simulink model "EMPlanner_cs"  (R2023a)
settings: Solver=ode5  StartTime=0.0  StopTime=60  FixedStep=1/1000  RelTol=1e-3
PreLoadFcn:
  | mbxruntime.callbacks.PreLoadFcn(bdroot);
PostLoadFcn:
  | mbxruntime.callbacks.PostLoadFcn(bdroot);
InitFcn:
  | mbxruntime.callbacks.InitFcn(bdroot);
StartFcn:
  | mbxruntime.callbacks.StartFcn(bdroot);
StopFcn:
  | mbxruntime.callbacks.StopFcn(bdroot);
model workspace: external: MAT-File .\EMPlanner_cs_hws.mat (data not in the file)
values from neighbouring files (symbols this model uses):
  c_factor = 43.75    [emplanner_init.m]
  cf = -64276.3    [emplanner_init.m]
  cr = -64276.3    [emplanner_init.m]
  KD_PID_distance = 0.0    (= 0)    [emplanner_init.m]
  KD_PID_speed = 0    [emplanner_init.m]
  KI_PID_distance = 0.0    (= 0)    [emplanner_init.m]
  KI_PID_speed = 0    [emplanner_init.m]
  KP_PID_distance = 0.5    [emplanner_init.m]
  KP_PID_speed = 1.8    [emplanner_init.m]
  la = 0.5989    [emplanner_init.m]
  lb = 1.1979-0.5989    (= 0.599)    [emplanner_init.m]
  LQR_K1 = k(:,1)'    [emplanner_init.m]
  LQR_K2 = k(:,2)'    [emplanner_init.m]
  LQR_K3 = k(:,3)'    [emplanner_init.m]
  LQR_K4 = k(:,4)'    [emplanner_init.m]
  m = 375.8    [emplanner_init.m]
  vx_break_point = zeros(1,5000)    [emplanner_init.m]
undefined symbols (not defined in the file or in its folder): aubr, DiscIntNeverNeededParam, EMPlanner_cs_27357ced727cddc2, EMPlanner_cs_3a309230b46bf2dd, EMPlanner_cs_4725e6271df7126f, EMPlanner_cs_7cd0898d5750b5ce, EMPlanner_cs_9531ed1ae61b92f2, EMPlanner_cs_Box_10_Dynamics_Empty_STATE_Box_10_Pitch0, EMPlanner_cs_Box_10_Dynamics_Empty_STATE_Box_10_Roll0, EMPlanner_cs_Box_10_Dynamics_Empty_STATE_Box_10_x0, EMPlanner_cs_Box_10_Dynamics_Empty_STATE_Box_10_y0, EMPlanner_cs_Box_10_Dynamics_Empty_STATE_Box_10_Yaw0, EMPlanner_cs_Box_10_Dynamics_Empty_STATE_Box_10_z0, EMPlanner_cs_Box_11_Dynamics_Empty_STATE_Box_11_Pitch0, EMPlanner_cs_Box_11_Dynamics_Empty_STATE_Box_11_Roll0, EMPlanner_cs_Box_11_Dynamics_Empty_STATE_Box_11_x0, EMPlanner_cs_Box_11_Dynamics_Empty_STATE_Box_11_y0, EMPlanner_cs_Box_11_Dynamics_Empty_STATE_Box_11_Yaw0, EMPlanner_cs_Box_11_Dynamics_Empty_STATE_Box_11_z0, EMPlanner_cs_Box_12_Dynamics_Empty_STATE_Box_12_Pitch0, EMPlanner_cs_Box_12_Dynamics_Empty_STATE_Box_12_Roll0, EMPlanner_cs_Box_12_Dynamics_Empty_STATE_Box_12_x0, EMPlanner_cs_Box_12_Dynamics_Empty_STATE_Box_12_y0, EMPlanner_cs_Box_12_Dynamics_Empty_STATE_Box_12_Yaw0, EMPlanner_cs_Box_12_Dynamics_Empty_STATE_Box_12_z0, EMPlanner_cs_Box_1_Path_pathUniqueID, EMPlanner_cs_Box_1_SpeedProfile_speedProfileUniqueID, EMPlanner_cs_Box_2_Path_pathUniqueID, EMPlanner_cs_Box_2_SpeedProfile_speedProfileUniqueID, EMPlanner_cs_Box_3_Path_pathUniqueID, EMPlanner_cs_Box_3_SpeedProfile_speedProfileUniqueID, EMPlanner_cs_Box_4_Path_pathUniqueID, EMPlanner_cs_Box_4_SpeedProfile_speedProfileUniqueID, EMPlanner_cs_Box_5_Dynamics_Empty_STATE_Box_5_Pitch0, EMPlanner_cs_Box_5_Dynamics_Empty_STATE_Box_5_Roll0, EMPlanner_cs_Box_5_Dynamics_Empty_STATE_Box_5_x0, EMPlanner_cs_Box_5_Dynamics_Empty_STATE_Box_5_y0, EMPlanner_cs_Box_5_Dynamics_Empty_STATE_Box_5_Yaw0, EMPlanner_cs_Box_5_Dynamics_Empty_STATE_Box_5_z0, EMPlanner_cs_Box_6_Path_pathUniqueID, EMPlanner_cs_Box_6_SpeedProfile_speedProfileUniqueID, EMPlanner_cs_Box_7_Dynamics_Empty_STATE_Box_7_Pitch0, EMPlanner_cs_Box_7_Dynamics_Empty_STATE_Box_7_Roll0, EMPlanner_cs_Box_7_Dynamics_Empty_STATE_Box_7_x0, EMPlanner_cs_Box_7_Dynamics_Empty_STATE_Box_7_y0, EMPlanner_cs_Box_7_Dynamics_Empty_STATE_Box_7_Yaw0, EMPlanner_cs_Box_7_Dynamics_Empty_STATE_Box_7_z0, EMPlanner_cs_Box_8_Dynamics_Empty_STATE_Box_8_Pitch0, EMPlanner_cs_Box_8_Dynamics_Empty_STATE_Box_8_Roll0, EMPlanner_cs_Box_8_Dynamics_Empty_STATE_Box_8_x0, EMPlanner_cs_Box_8_Dynamics_Empty_STATE_Box_8_y0, EMPlanner_cs_Box_8_Dynamics_Empty_STATE_Box_8_Yaw0, EMPlanner_cs_Box_8_Dynamics_Empty_STATE_Box_8_z0, EMPlanner_cs_Box_9_Dynamics_Empty_STATE_Box_9_Pitch0, EMPlanner_cs_Box_9_Dynamics_Empty_STATE_Box_9_Roll0, EMPlanner_cs_Box_9_Dynamics_Empty_STATE_Box_9_x0, EMPlanner_cs_Box_9_Dynamics_Empty_STATE_Box_9_y0, EMPlanner_cs_Box_9_Dynamics_Empty_STATE_Box_9_Yaw0, EMPlanner_cs_Box_9_Dynamics_Empty_STATE_Box_9_z0, EMPlanner_cs_dca7ae789a013f83 ... (+7)
libraries: PreScanSimulinkLibrary x16, Solver_SF x1
(part 7 of 10)

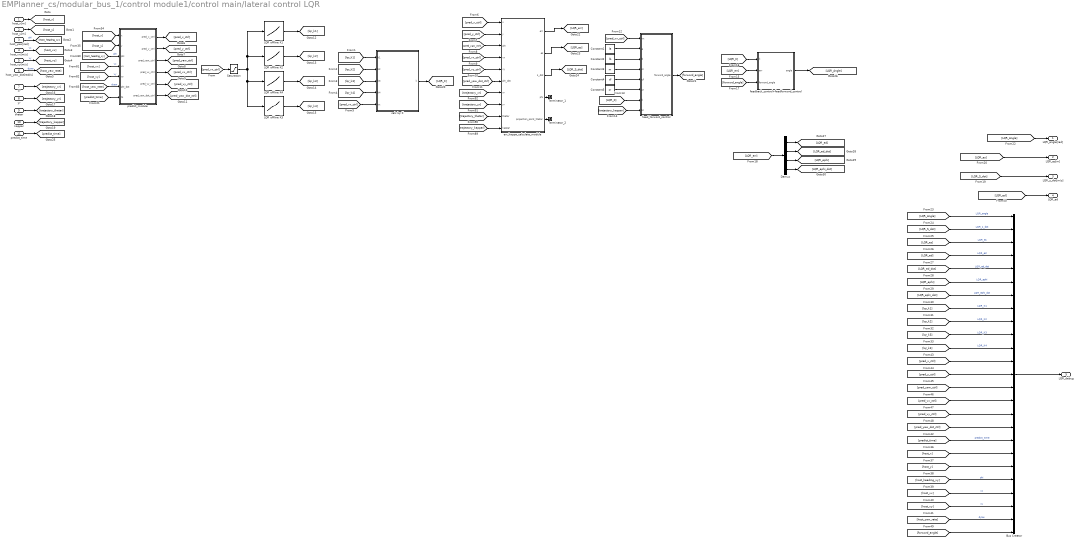
== system EMPlanner_cs/modular_bus_1/control module1/control main/lateral control LQR ==
  host_x[m] : Inport
  host_y[m] : Inport  Port=2
  host_yaw[rad] : Inport  Port=3
  host_vx[m/s] : Inport  Port=4
  host_vy[m/s] : Inport  Port=5
  host_yaw_dot[rad/s] : Inport  Port=6
  xr : Inport  Port=7
  yr : Inport  Port=8
  thetar : Inport  Port=9
  kappar : Inport  Port=10
  predict_time : Inport  Port=11
  Bus Creator : BusCreator  Inputs=25
  Constant1 : Constant  Value=la
  Constant2 : Constant  Value=lb
  Constant3 : Constant  Value=m
  Constant4 : Constant  Value=cf
  Constant5 : Constant  Value=cr
  Demux : Demux
  LQR offline K1 : Lookup_n-D  NumberOfTableDimensions=1  BreakpointsForDimension1=vx_break_point  Table=LQR_K1  InternalRulePriority=Speed  RndMeth=Simplest
  LQR offline K2 : Lookup_n-D  NumberOfTableDimensions=1  BreakpointsForDimension1=vx_break_point  Table=LQR_K2  InternalRulePriority=Speed  RndMeth=Simplest
  LQR offline K3 : Lookup_n-D  NumberOfTableDimensions=1  BreakpointsForDimension1=vx_break_point  Table=LQR_K3  InternalRulePriority=Speed  RndMeth=Simplest
  LQR offline K4 : Lookup_n-D  NumberOfTableDimensions=1  BreakpointsForDimension1=vx_break_point  Table=LQR_K4  InternalRulePriority=Speed  RndMeth=Simplest
  Saturation : Saturate  UpperLimit=50  LowerLimit=0
  Terminator_1 : Terminator
  Terminator_2 : Terminator
  calc lqr K : MATLAB Function  TreatAsAtomicUnit=on
  err_kappa_calculate_module : MATLAB Function  TreatAsAtomicUnit=on
  feed_forword_control : MATLAB Function  TreatAsAtomicUnit=on
  feedback_control+feedforword_control : MATLAB Function  TreatAsAtomicUnit=on
  predict_module : MATLAB Function  TreatAsAtomicUnit=on
  LQR_angle[rad] : Outport  VectorParamsAs1DForOutWhenUnconnected=off
  LQR_es[m] : Outport  Port=2  VectorParamsAs1DForOutWhenUnconnected=off
  LQR_s_dot[m/s] : Outport  Port=3  VectorParamsAs1DForOutWhenUnconnected=off
  LQR_ed : Outport  Port=4  VectorParamsAs1DForOutWhenUnconnected=off
  LQR_debug : Outport  Port=5  VectorParamsAs1DForOutWhenUnconnected=off
  wires:
  err_kappa_calculate_module/5(projection_point_thetar) -> Terminator_2/1
  err_kappa_calculate_module/4(phi) -> Terminator_1/1
  [LQR_ed] -> LQR_ed/1
  [forword_angle] -> Bus Creator/25
  [host_yaw_rate] -> Bus Creator/24  "dyaw"
  [host_vy] -> Bus Creator/23  "vy"
  [host_vx] -> Bus Creator/22  "vx"
  [host_heading_xy] -> Bus Creator/21  "phi"
  [host_y] -> Bus Creator/20
  [host_x] -> Bus Creator/19
  [predict_time] -> Bus Creator/18  "predict_time"
  [pred_yaw_dot_ctrl] -> Bus Creator/17
  [pred_vy_ctrl] -> Bus Creator/16
  [pred_vx_ctrl] -> Bus Creator/15
  [pred_yaw_ctrl] -> Bus Creator/14
  [pred_y_ctrl] -> Bus Creator/13
  [pred_x_ctrl] -> Bus Creator/12
  [lqr_k4] -> Bus Creator/11  "LQR_K4"
  [lqr_k3] -> Bus Creator/10  "LQR_K3"
  [lqr_k2] -> Bus Creator/9  "LQR_K2"
  [lqr_k1] -> Bus Creator/8  "LQR_K1"
  [LQR_ephi_dot] -> Bus Creator/7  "LQR_ephi_dot"
  [LQR_ephi] -> Bus Creator/6  "LQR_ephi"
  [LQR_ed_dot] -> Bus Creator/5  "LQR_ed_dot"
  [LQR_ed] -> Bus Creator/4  "LQR_ed"
  Demux/4 -> [LQR_ephi_dot]
  Demux/3 -> [LQR_ephi]
  Demux/2 -> [LQR_ed_dot]
  Demux/1 -> [LQR_ed]
  [LQR_es] -> Bus Creator/3  "LQR_es"
  [LQR_S_dot] -> Bus Creator/2  "LQR_s_dot"
  [LQR_Angle] -> Bus Creator/1  "LQR_angle"
  [LQR_Angle] -> LQR_angle[rad]/1
  feedback_control+feedforword_control/1(angle) -> [LQR_Angle]
  Bus Creator/1 -> LQR_debug/1
  predict_time/1 -> [predict_time]
  Saturation/1 -> LQR offline K1/1, LQR offline K2/1, LQR offline K4/1, LQR offline K3/1
  [LQR_es] -> LQR_es[m]/1
  [LQR_S_dot] -> LQR_s_dot[m/s]/1
  err_kappa_calculate_module/3(s_dot) -> [LQR_S_dot]
  err_kappa_calculate_module/2(es) -> [LQR_es]
  [LQR_err] -> Demux/1
  [forword_angle] -> feedback_control+feedforword_control/3(forword_angle)
  [LQR_K] -> feedback_control+feedforword_control/1(k)
  [LQR_err] -> feedback_control+feedforword_control/2(err)
  err_kappa_calculate_module/1(err) -> [LQR_err]
  feed_forword_control/1(forword_angle) -> [forword_angle]
  [trajectory_kappar] -> feed_forword_control/8(kr)
  [LQR_K] -> feed_forword_control/7(k)
  calc lqr K/1(k) -> [LQR_K]
  Constant5/1 -> feed_forword_control/6(cr)
  Constant4/1 -> feed_forword_control/5(cf)
  Constant3/1 -> feed_forword_control/4(m)
  Constant2/1 -> feed_forword_control/3(b)
  Constant1/1 -> feed_forword_control/2(a)
  [pred_vx_ctrl] -> feed_forword_control/1(vx)
  [trajectory_thetar] -> err_kappa_calculate_module/9(thetar)
  [trajectory_kappar] -> err_kappa_calculate_module/10(kappar)
  [trajectory_yr] -> err_kappa_calculate_module/8(yr)
  [trajectory_xr] -> err_kappa_calculate_module/7(xr)
  kappar/1 -> [trajectory_kappar]
  thetar/1 -> [trajectory_thetar]
  yr/1 -> [trajectory_yr]
  xr/1 -> [trajectory_xr]
  [pred_yaw_dot_ctrl] -> err_kappa_calculate_module/6(phi_dot)
  [pred_vy_ctrl] -> err_kappa_calculate_module/5(vy)
  [pred_vx_ctrl] -> err_kappa_calculate_module/4(vx)
  [pred_yaw_ctrl] -> err_kappa_calculate_module/3("phi ")
  [pred_y_ctrl] -> err_kappa_calculate_module/2(y)
  [pred_x_ctrl] -> err_kappa_calculate_module/1(x)
  [lqr_k1] -> calc lqr K/1(k1)
  [lqr_k2] -> calc lqr K/2(k2)
  [lqr_k3] -> calc lqr K/3(k3)
  [lqr_k4] -> calc lqr K/4(k4)
  [pred_vx_ctrl] -> calc lqr K/5(vx)
  LQR offline K3/1 -> [lqr_k4]
  LQR offline K4/1 -> [lqr_k3]
  LQR offline K2/1 -> [lqr_k2]
  LQR offline K1/1 -> [lqr_k1]
  [pred_vx_ctrl] -> Saturation/1
  predict_module/6(pred_yaw_dot_ctrl) -> [pred_yaw_dot_ctrl]
  predict_module/5(pred_vy_ctrl) -> [pred_vy_ctrl]
  predict_module/4(pred_vx_ctrl) -> [pred_vx_ctrl]
  predict_module/3(pred_yaw_ctrl) -> [pred_yaw_ctrl]
  predict_module/2(pred_y_ctrl) -> [pred_y_ctrl]
  predict_module/1(pred_x_ctrl) -> [pred_x_ctrl]
  host_yaw_dot[rad/s]/1 -> [host_yaw_rate]  "dyaw"
  host_vy[m/s]/1 -> [host_vy]  "vy"
  host_vx[m/s]/1 -> [host_vx]  "vx"
  host_yaw[rad]/1 -> [host_heading_xy]  "phi"
  host_y[m]/1 -> [host_y]
  host_x[m]/1 -> [host_x]
  [predict_time] -> predict_module/7(ts)
  [host_heading_xy] -> predict_module/3(phi)  "phi"
  [host_y] -> predict_module/2(y)
  [host_vx] -> predict_module/4(vx)  "vx"
  [host_yaw_rate] -> predict_module/6(phi_dot)  "dyaw"
  [host_x] -> predict_module/1(x)
  [host_vy] -> predict_module/5(vy)  "vy"

== system EMPlanner_cs/modular_bus_1/control module1/control main/longitudinal control double PID ==
  s_err[m] : Inport
  speed_desire[m/s] : Inport  Port=2
  accelerate desire[m/s^2] : Inport  Port=3
  host_speed[m/s] : Inport  Port=4
  host_s_dot[m/s] : Inport  Port=5
  KP_PID_distance : Inport  Port=6
  KI_PID_distance : Inport  Port=7
  KD_PID_distance : Inport  Port=8
  KP_PID_speed : Inport  Port=9
  KI_PID_speed : Inport  Port=10
  KD_PID_speed : Inport  Port=11
  2-D Lookup Table : Lookup_n-D  BreakpointsForDimension1=vubr  BreakpointsForDimension2=aubr  Table=tablebr  InternalRulePriority=Speed  RndMeth=Simplest
      settings: InputPortMap=u0,u1
  Add : Sum  Inputs=++-
  Add1 : Sum
  Bus Creator : BusCreator  Inputs=9
  Discrete Filter : DiscreteFilter
  MATLAB Function1 : MATLAB Function  TreatAsAtomicUnit=on
  Saturation : Saturate  UpperLimit=45  LowerLimit=-45
  Saturation1 : Saturate  UpperLimit=5  LowerLimit=-8
  discrete pid distance : Subsystem
  discrete pid speed : Subsystem
  throttle : Outport
  brake : Outport  Port=2
  longitudinal_debug : Outport  Port=3
  wires:
  discrete pid distance/1(pid_out) -> Add/1
  [KD_PID_speed] -> discrete pid speed/4(kd)
  [KI_PID_speed] -> discrete pid speed/3(ki)
  [KP_PID_speed] -> discrete pid speed/2(kp)
  [KD_PID_distance] -> discrete pid distance/4(kd)
  [KI_PID_distance] -> discrete pid distance/3(ki)
  [KP_PID_distance] -> discrete pid distance/2(kp)
  Discrete Filter/1 -> discrete pid distance/1(err)
  Bus Creator/1 -> longitudinal_debug/1
  [host_s_dot] -> Bus Creator/9  "host_s_dot"
  [s_err] -> Bus Creator/8  "s_err"
  [host_speed] -> Bus Creator/7  "host_speed"
  [KD_PID_speed] -> Bus Creator/6  "KD_PID_speed"
  [KI_PID_speed] -> Bus Creator/5  "KI_PID_speed"
  [KP_PID_speed] -> Bus Creator/4  "KP_PID_speed"
  [KD_PID_distance] -> Bus Creator/3  "KD_PID_distance"
  [KI_PID_distance] -> Bus Creator/2  "KI_PID_distance"
  [KP_PID_distance] -> Bus Creator/1  "KP_PID_distance"
  MATLAB Function1/2(brake) -> brake/1
  MATLAB Function1/1(throttle) -> throttle/1
  [host_speed] -> 2-D Lookup Table/1
  [host_s_dot] -> Add/3
  host_s_dot[m/s]/1 -> [host_s_dot]
  Saturation1/1 -> 2-D Lookup Table/2
  Add1/1 -> Saturation1/1
  [accelerate_desire] -> Add1/2
  discrete pid speed/1(pid_out) -> Add1/1
  Saturation/1 -> discrete pid speed/1(err)
  Add/1 -> Saturation/1
  [speed_desire] -> Add/2
  host_speed[m/s]/1 -> [host_speed]
  [s_err] -> Discrete Filter/1
  KD_PID_speed/1 -> [KD_PID_speed]
  KI_PID_speed/1 -> [KI_PID_speed]
  KP_PID_speed/1 -> [KP_PID_speed]
  KD_PID_distance/1 -> [KD_PID_distance]
  KI_PID_distance/1 -> [KI_PID_distance]
  KP_PID_distance/1 -> [KP_PID_distance]
  accelerate desire[m/s^2]/1 -> [accelerate_desire]
  speed_desire[m/s]/1 -> [speed_desire]
  s_err[m]/1 -> [s_err]
  2-D Lookup Table/1 -> MATLAB Function1/1(u)

== system EMPlanner_cs/modular_bus_1/control module1/control main/understeer compensate ==
  LQR_angle : Inport
  lateral err : Inport  Port=2
  Add : Sum  Inputs=+-
  Gain : Gain  Gain=0.01
  Manual Switch : ManualSwitch
  LQR_final_angle : Outport
  wires:
  Gain/1 -> Add/2
  LQR_angle/1 -> Manual Switch/1, Add/1
  Manual Switch/1 -> LQR_final_angle/1
  Add/1 -> Manual Switch/2
  lateral err/1 -> Gain/1

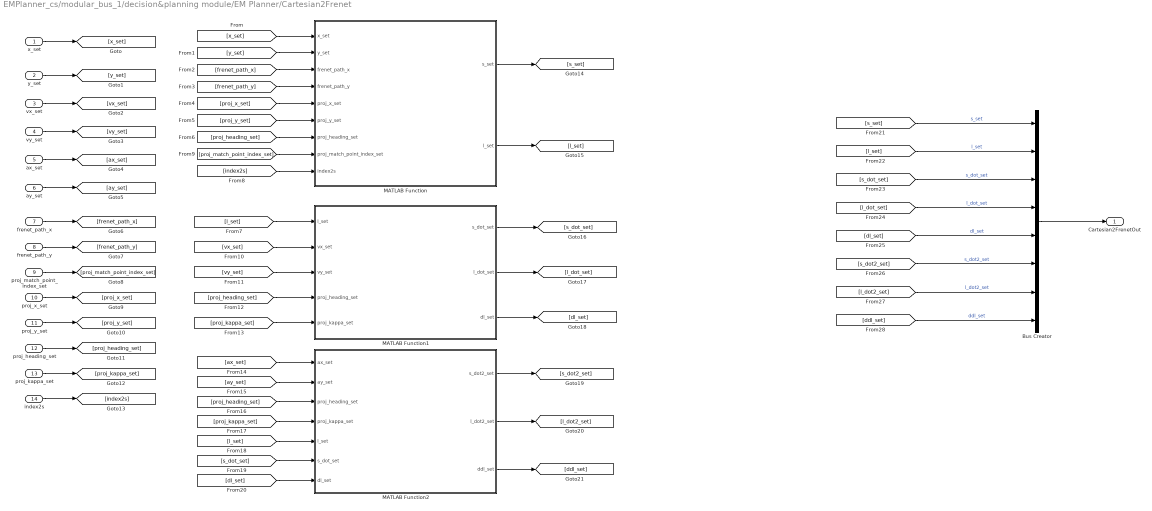
== system EMPlanner_cs/modular_bus_1/decision&planning module/EM Planner/Cartesian2Frenet ==
  x_set : Inport
  y_set : Inport  Port=2
  vx_set : Inport  Port=3
  vy_set : Inport  Port=4
  ax_set : Inport  Port=5
  ay_set : Inport  Port=6
  frenet_path_x : Inport  Port=7
  frenet_path_y : Inport  Port=8
  proj_match_point_index_set : Inport  Port=9
  proj_x_set : Inport  Port=10
  proj_y_set : Inport  Port=11
  proj_heading_set : Inport  Port=12
  proj_kappa_set : Inport  Port=13
  index2s : Inport  Port=14
  Bus Creator : BusCreator  Inputs=8
  MATLAB Function : MATLAB Function  TreatAsAtomicUnit=on
  MATLAB Function1 : MATLAB Function  TreatAsAtomicUnit=on
  MATLAB Function2 : MATLAB Function  TreatAsAtomicUnit=on
  Cartesian2FrenetOut : Outport
  wires:
  Bus Creator/1 -> Cartesian2FrenetOut/1
  [ddl_set] -> Bus Creator/8  "ddl_set"
  [l_dot2_set] -> Bus Creator/7  "l_dot2_set"
  [s_dot2_set] -> Bus Creator/6  "s_dot2_set"
  [dl_set] -> Bus Creator/5  "dl_set"
  [l_dot_set] -> Bus Creator/4  "l_dot_set"
  [s_dot_set] -> Bus Creator/3  "s_dot_set"
  [l_set] -> Bus Creator/2  "l_set"
  [s_set] -> Bus Creator/1  "s_set"
  MATLAB Function2/3(ddl_set) -> [ddl_set]
  MATLAB Function2/2(l_dot2_set) -> [l_dot2_set]
  MATLAB Function2/1(s_dot2_set) -> [s_dot2_set]
  [dl_set] -> MATLAB Function2/7(dl_set)
  [s_dot_set] -> MATLAB Function2/6(s_dot_set)
  MATLAB Function1/3(dl_set) -> [dl_set]
  MATLAB Function1/2(l_dot_set) -> [l_dot_set]
  MATLAB Function1/1(s_dot_set) -> [s_dot_set]
  [l_set] -> MATLAB Function2/5(l_set)
  [proj_kappa_set] -> MATLAB Function2/4(proj_kappa_set)
  [proj_heading_set] -> MATLAB Function2/3(proj_heading_set)
  [ay_set] -> MATLAB Function2/2(ay_set)
  [ax_set] -> MATLAB Function2/1(ax_set)
  [proj_kappa_set] -> MATLAB Function1/5(proj_kappa_set)
  [proj_heading_set] -> MATLAB Function1/4(proj_heading_set)
  [vy_set] -> MATLAB Function1/3(vy_set)
  [vx_set] -> MATLAB Function1/2(vx_set)
  [l_set] -> MATLAB Function1/1(l_set)
  MATLAB Function/2(l_set) -> [l_set]
  MATLAB Function/1(s_set) -> [s_set]
  [index2s] -> MATLAB Function/9(index2s)
  [proj_heading_set] -> MATLAB Function/7(proj_heading_set)
  [proj_y_set] -> MATLAB Function/6(proj_y_set)
  [proj_match_point_index_set] -> MATLAB Function/8(proj_match_point_index_set)
  [proj_x_set] -> MATLAB Function/5(proj_x_set)
  [frenet_path_y] -> MATLAB Function/4(frenet_path_y)
  [frenet_path_x] -> MATLAB Function/3(frenet_path_x)
  [y_set] -> MATLAB Function/2(y_set)
  [x_set] -> MATLAB Function/1(x_set)
  index2s/1 -> [index2s]
  proj_kappa_set/1 -> [proj_kappa_set]
  proj_heading_set/1 -> [proj_heading_set]
  proj_y_set/1 -> [proj_y_set]
  proj_x_set/1 -> [proj_x_set]
  proj_match_point_index_set/1 -> [proj_match_point_index_set]
  frenet_path_y/1 -> [frenet_path_y]
  frenet_path_x/1 -> [frenet_path_x]
  ay_set/1 -> [ay_set]
  ax_set/1 -> [ax_set]
  vy_set/1 -> [vy_set]
  vx_set/1 -> [vx_set]
  y_set/1 -> [y_set]
  x_set/1 -> [x_set]

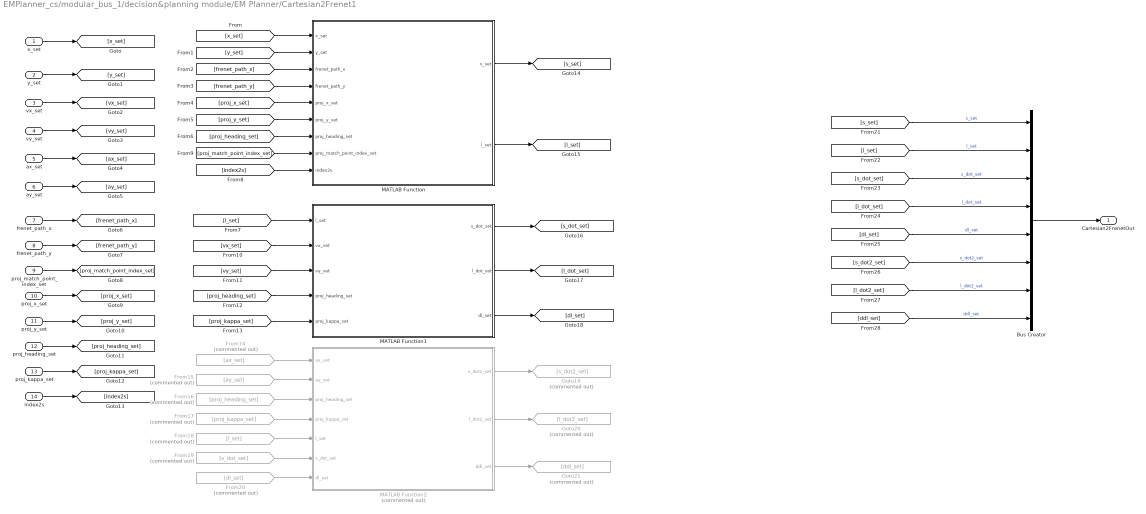
== system EMPlanner_cs/modular_bus_1/decision&planning module/EM Planner/Cartesian2Frenet1 ==
  x_set : Inport
  y_set : Inport  Port=2
  vx_set : Inport  Port=3
  vy_set : Inport  Port=4
  ax_set : Inport  Port=5
  ay_set : Inport  Port=6
  frenet_path_x : Inport  Port=7
  frenet_path_y : Inport  Port=8
  proj_match_point_index_set : Inport  Port=9
  proj_x_set : Inport  Port=10
  proj_y_set : Inport  Port=11
  proj_heading_set : Inport  Port=12
  proj_kappa_set : Inport  Port=13
  index2s : Inport  Port=14
  Bus Creator : BusCreator  Inputs=8
  From14 : From  Commented=on  GotoTag=ax_set
  From15 : From  Commented=on  GotoTag=ay_set
  From16 : From  Commented=on  GotoTag=proj_heading_set
  From17 : From  Commented=on  GotoTag=proj_kappa_set
  From18 : From  Commented=on  GotoTag=l_set
  From19 : From  Commented=on  GotoTag=s_dot_set
  From20 : From  Commented=on  GotoTag=dl_set
  Goto19 : Goto  Commented=on  GotoTag=s_dot2_set
  Goto20 : Goto  Commented=on  GotoTag=l_dot2_set
  Goto21 : Goto  Commented=on  GotoTag=ddl_set
  MATLAB Function : MATLAB Function  TreatAsAtomicUnit=on
  MATLAB Function1 : MATLAB Function  TreatAsAtomicUnit=on
  MATLAB Function2 : MATLAB Function  Commented=on  TreatAsAtomicUnit=on
  Cartesian2FrenetOut : Outport
  wires:
  x_set/1 -> [x_set]
  y_set/1 -> [y_set]
  vx_set/1 -> [vx_set]
  vy_set/1 -> [vy_set]
  ax_set/1 -> [ax_set]
  ay_set/1 -> [ay_set]
  frenet_path_x/1 -> [frenet_path_x]
  frenet_path_y/1 -> [frenet_path_y]
  proj_match_point_index_set/1 -> [proj_match_point_index_set]
  proj_x_set/1 -> [proj_x_set]
  proj_y_set/1 -> [proj_y_set]
  proj_heading_set/1 -> [proj_heading_set]
  proj_kappa_set/1 -> [proj_kappa_set]
  index2s/1 -> [index2s]
  [x_set] -> MATLAB Function/1(x_set)
  [y_set] -> MATLAB Function/2(y_set)
  [frenet_path_x] -> MATLAB Function/3(frenet_path_x)
  [frenet_path_y] -> MATLAB Function/4(frenet_path_y)
  [proj_x_set] -> MATLAB Function/5(proj_x_set)
  [proj_match_point_index_set] -> MATLAB Function/8(proj_match_point_index_set)
  [proj_y_set] -> MATLAB Function/6(proj_y_set)
  [proj_heading_set] -> MATLAB Function/7(proj_heading_set)
  [index2s] -> MATLAB Function/9(index2s)
  MATLAB Function/1(s_set) -> [s_set]
  MATLAB Function/2(l_set) -> [l_set]
  [l_set] -> MATLAB Function1/1(l_set)
  [vx_set] -> MATLAB Function1/2(vx_set)
  [vy_set] -> MATLAB Function1/3(vy_set)
  [proj_heading_set] -> MATLAB Function1/4(proj_heading_set)
  [proj_kappa_set] -> MATLAB Function1/5(proj_kappa_set)
  From14/1 -> MATLAB Function2/1(ax_set)
  From15/1 -> MATLAB Function2/2(ay_set)
  From16/1 -> MATLAB Function2/3(proj_heading_set)
  From17/1 -> MATLAB Function2/4(proj_kappa_set)
  From18/1 -> MATLAB Function2/5(l_set)
  MATLAB Function1/1(s_dot_set) -> [s_dot_set]
  MATLAB Function1/2(l_dot_set) -> [l_dot_set]
  MATLAB Function1/3(dl_set) -> [dl_set]
  From19/1 -> MATLAB Function2/6(s_dot_set)
  From20/1 -> MATLAB Function2/7(dl_set)
  MATLAB Function2/1(s_dot2_set) -> Goto19/1
  MATLAB Function2/2(l_dot2_set) -> Goto20/1
  MATLAB Function2/3(ddl_set) -> Goto21/1
  [s_set] -> Bus Creator/1  "s_set"
  [l_set] -> Bus Creator/2  "l_set"
  [s_dot_set] -> Bus Creator/3  "s_dot_set"
  [l_dot_set] -> Bus Creator/4  "l_dot_set"
  [dl_set] -> Bus Creator/5  "dl_set"
  [s_dot2_set] -> Bus Creator/6  "s_dot2_set"
  [l_dot2_set] -> Bus Creator/7  "l_dot2_set"
  [ddl_set] -> Bus Creator/8  "ddl_set"
  Bus Creator/1 -> Cartesian2FrenetOut/1

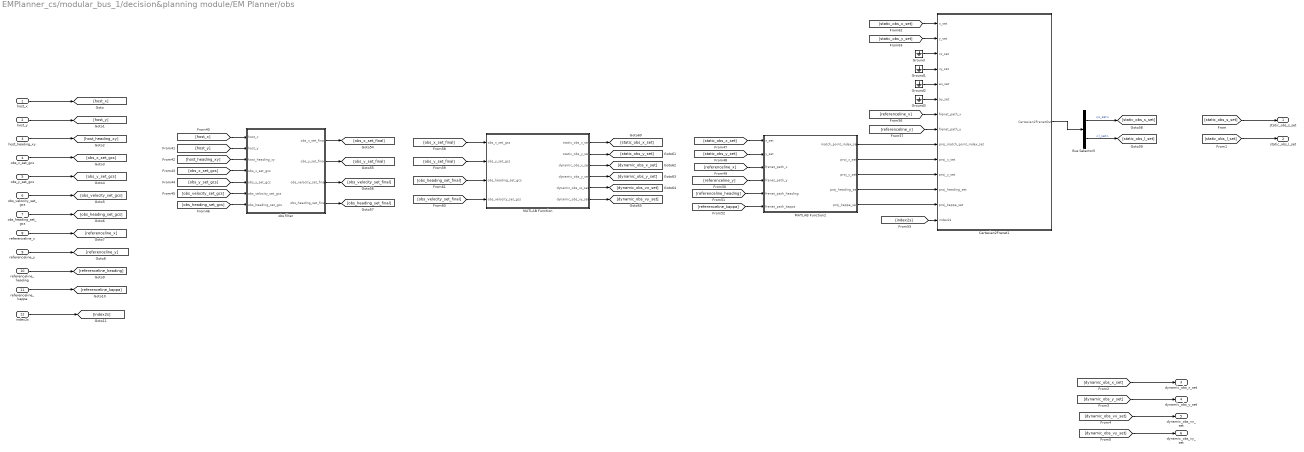
== system EMPlanner_cs/modular_bus_1/decision&planning module/EM Planner/obs ==
  host_x : Inport
  host_y : Inport  Port=2
  host_heading_xy : Inport  Port=3
  obs_x_set_gcs : Inport  Port=4
  obs_y_set_gcs : Inport  Port=5
  obs_velocity_set_gcs : Inport  Port=6
  obs_heading_set_gcs : Inport  Port=7
  referenceline_x : Inport  Port=8
  referenceline_y : Inport  Port=9
  referenceline_heading : Inport  Port=10
  referenceline_kappa : Inport  Port=11
  index2s : Inport  Port=12
  Bus Selector5 : BusSelector  OutputSignals=s_set,l_set
  Cartesian2Frenet1 : Subsystem
  Ground{,1..3} (4 alike) : Ground
  MATLAB Function : MATLAB Function  TreatAsAtomicUnit=on
  MATLAB Function2 : MATLAB Function  TreatAsAtomicUnit=on
  obs filter : MATLAB Function  TreatAsAtomicUnit=on
  static_obs_s_set : Outport
  static_obs_l_set : Outport  Port=2
  dynamic_obs_x_set : Outport  Port=3
  dynamic_obs_y_set : Outport  Port=4
  dynamic_obs_vx_set : Outport  Port=5
  dynamic_obs_vy_set : Outport  Port=6
  wires:
  [obs_heading_set_final] -> MATLAB Function/3(obs_heading_set_gcs)
  [obs_velocity_set_final] -> MATLAB Function/4(obs_velocity_set_gcs)
  [dynamic_obs_x_set] -> dynamic_obs_x_set/1
  [dynamic_obs_y_set] -> dynamic_obs_y_set/1
  [dynamic_obs_vx_set] -> dynamic_obs_vx_set/1
  [dynamic_obs_vy_set] -> dynamic_obs_vy_set/1
  [static_obs_l_set] -> static_obs_l_set/1
  [static_obs_s_set] -> static_obs_s_set/1
  index2s/1 -> [index2s]
  referenceline_kappa/1 -> [referenceline_kappa]
  referenceline_heading/1 -> [referenceline_heading]
  referenceline_y/1 -> [referenceline_y]
  referenceline_x/1 -> [referenceline_x]
  obs_heading_set_gcs/1 -> [obs_heading_set_gcs]
  obs_velocity_set_gcs/1 -> [obs_velocity_set_gcs]
  obs_y_set_gcs/1 -> [obs_y_set_gcs]
  obs_x_set_gcs/1 -> [obs_x_set_gcs]
  host_heading_xy/1 -> [host_heading_xy]
  host_y/1 -> [host_y]
  host_x/1 -> [host_x]
  [static_obs_y_set] -> Cartesian2Frenet1/2(y_set)
  MATLAB Function/2(static_obs_y_set) -> [static_obs_y_set]
  [static_obs_x_set] -> MATLAB Function2/1(x_set)
  Cartesian2Frenet1/1(Cartesian2FrenetOut) -> Bus Selector5/1
  [obs_y_set_gcs] -> obs filter/5(obs_y_set_gcs)
  [host_x] -> obs filter/1(host_x)
  MATLAB Function2/1(match_point_index_set) -> Cartesian2Frenet1/9(proj_match_point_index_set)
  MATLAB Function/4(dynamic_obs_y_set) -> [dynamic_obs_y_set]
  MATLAB Function2/3(proj_y_set) -> Cartesian2Frenet1/11(proj_y_set)
  Ground/1 -> Cartesian2Frenet1/3(vx_set)
  MATLAB Function2/2(proj_x_set) -> Cartesian2Frenet1/10(proj_x_set)
  MATLAB Function/3(dynamic_obs_x_set) -> [dynamic_obs_x_set]
  Bus Selector5/1 -> [static_obs_s_set]  "<s_set>"
  obs filter/2(obs_y_set_final) -> [obs_y_set_final]
  [referenceline_heading] -> MATLAB Function2/5(frenet_path_heading)
  Bus Selector5/2 -> [static_obs_l_set]  "<l_set>"
  [host_y] -> obs filter/2(host_y)
  [obs_velocity_set_gcs] -> obs filter/6(obs_velocity_set_gcs)
  [obs_x_set_final] -> MATLAB Function/1(obs_x_set_gcs)
  Ground1/1 -> Cartesian2Frenet1/4(vy_set)
  [referenceline_x] -> Cartesian2Frenet1/7(frenet_path_x)
  [static_obs_y_set] -> MATLAB Function2/2(y_set)
  [static_obs_x_set] -> Cartesian2Frenet1/1(x_set)
  [referenceline_kappa] -> MATLAB Function2/6(frenet_path_kappa)
  [obs_heading_set_gcs] -> obs filter/7(obs_heading_set_gcs)
  MATLAB Function/1(static_obs_x_set) -> [static_obs_x_set]
  obs filter/3(obs_velocity_set_final) -> [obs_velocity_set_final]
  [referenceline_y] -> MATLAB Function2/4(frenet_path_y)
  MATLAB Function/6(dynamic_obs_vy_set) -> [dynamic_obs_vy_set]
  [obs_y_set_final] -> MATLAB Function/2(obs_y_set_gcs)
  MATLAB Function/5(dynamic_obs_vx_set) -> [dynamic_obs_vx_set]
  [host_heading_xy] -> obs filter/3(host_heading_xy)
  obs filter/4(obs_heading_set_final) -> [obs_heading_set_final]
  obs filter/1(obs_x_set_final) -> [obs_x_set_final]
  Ground2/1 -> Cartesian2Frenet1/5(ax_set)
  [referenceline_x] -> MATLAB Function2/3(frenet_path_x)
  MATLAB Function2/4(proj_heading_set) -> Cartesian2Frenet1/12(proj_heading_set)
  MATLAB Function2/5(proj_kappa_set) -> Cartesian2Frenet1/13(proj_kappa_set)
  [referenceline_y] -> Cartesian2Frenet1/8(frenet_path_y)
  [index2s] -> Cartesian2Frenet1/14(index2s)
  [obs_x_set_gcs] -> obs filter/4(obs_x_set_gcs)
  Ground3/1 -> Cartesian2Frenet1/6(ay_set)

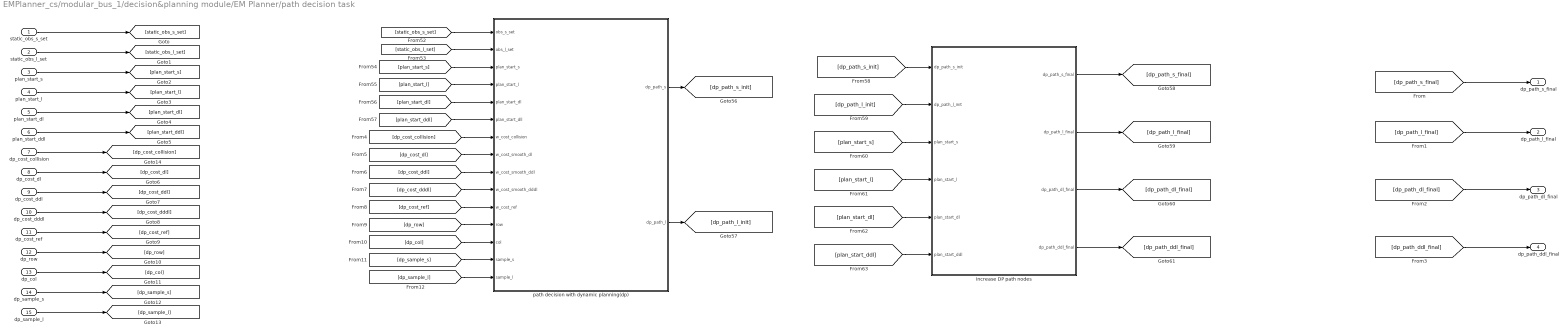
== system EMPlanner_cs/modular_bus_1/decision&planning module/EM Planner/path decision task ==
  static_obs_s_set : Inport
  static_obs_l_set : Inport  Port=2
  plan_start_s : Inport  Port=3
  plan_start_l : Inport  Port=4
  plan_start_dl : Inport  Port=5
  plan_start_ddl : Inport  Port=6
  dp_cost_collision : Inport  Port=7
  dp_cost_dl : Inport  Port=8
  dp_cost_ddl : Inport  Port=9
  dp_cost_dddl : Inport  Port=10
  dp_cost_ref : Inport  Port=11
  dp_row : Inport  Port=12
  dp_col : Inport  Port=13
  dp_sample_s : Inport  Port=14
  dp_sample_l : Inport  Port=15
  increase DP path nodes : MATLAB Function  TreatAsAtomicUnit=on
  path decision with dynamic planning(dp) : MATLAB Function  TreatAsAtomicUnit=on
  dp_path_s_final : Outport
  dp_path_l_final : Outport  Port=2
  dp_path_dl_final : Outport  Port=3
  dp_path_ddl_final : Outport  Port=4
  wires:
  dp_cost_collision/1 -> [dp_cost_collision]
  dp_sample_s/1 -> [dp_sample_s]
  dp_sample_l/1 -> [dp_sample_l]
  dp_col/1 -> [dp_col]
  dp_row/1 -> [dp_row]
  dp_cost_ref/1 -> [dp_cost_ref]
  dp_cost_dddl/1 -> [dp_cost_dddl]
  dp_cost_ddl/1 -> [dp_cost_ddl]
  dp_cost_dl/1 -> [dp_cost_dl]
  [dp_sample_l] -> path decision with dynamic planning(dp)/15(sample_l)
  [dp_sample_s] -> path decision with dynamic planning(dp)/14(sample_s)
  [dp_col] -> path decision with dynamic planning(dp)/13(col)
  [dp_row] -> path decision with dynamic planning(dp)/12(row)
  [dp_cost_ref] -> path decision with dynamic planning(dp)/11(w_cost_ref)
  [dp_cost_dddl] -> path decision with dynamic planning(dp)/10(w_cost_smooth_dddl)
  [dp_cost_ddl] -> path decision with dynamic planning(dp)/9(w_cost_smooth_ddl)
  [dp_cost_dl] -> path decision with dynamic planning(dp)/8(w_cost_smooth_dl)
  [dp_cost_collision] -> path decision with dynamic planning(dp)/7(w_cost_collision)
  [dp_path_ddl_final] -> dp_path_ddl_final/1
  [dp_path_dl_final] -> dp_path_dl_final/1
  [dp_path_l_final] -> dp_path_l_final/1
  [dp_path_s_final] -> dp_path_s_final/1
  plan_start_ddl/1 -> [plan_start_ddl]
  plan_start_dl/1 -> [plan_start_dl]
  plan_start_l/1 -> [plan_start_l]
  plan_start_s/1 -> [plan_start_s]
  static_obs_l_set/1 -> [static_obs_l_set]
  static_obs_s_set/1 -> [static_obs_s_set]
  [dp_path_s_init] -> increase DP path nodes/1(dp_path_s_init)
  [dp_path_l_init] -> increase DP path nodes/2(dp_path_l_init)
  [plan_start_s] -> increase DP path nodes/3(plan_start_s)
  [plan_start_dl] -> path decision with dynamic planning(dp)/5(plan_start_dl)
  [plan_start_ddl] -> increase DP path nodes/6(plan_start_ddl)
  [plan_start_l] -> increase DP path nodes/4(plan_start_l)
  path decision with dynamic planning(dp)/2(dp_path_l) -> [dp_path_l_init]
  increase DP path nodes/3(dp_path_dl_final) -> [dp_path_dl_final]
  increase DP path nodes/1(dp_path_s_final) -> [dp_path_s_final]
  increase DP path nodes/4(dp_path_ddl_final) -> [dp_path_ddl_final]
  [plan_start_dl] -> increase DP path nodes/5(plan_start_dl)
  [static_obs_s_set] -> path decision with dynamic planning(dp)/1(obs_s_set)
  [plan_start_l] -> path decision with dynamic planning(dp)/4(plan_start_l)
  [plan_start_ddl] -> path decision with dynamic planning(dp)/6(plan_start_dll)
  [static_obs_l_set] -> path decision with dynamic planning(dp)/2(obs_l_set)
  increase DP path nodes/2(dp_path_l_final) -> [dp_path_l_final]
  path decision with dynamic planning(dp)/1(dp_path_s) -> [dp_path_s_init]
  [plan_start_s] -> path decision with dynamic planning(dp)/3(plan_start_s)

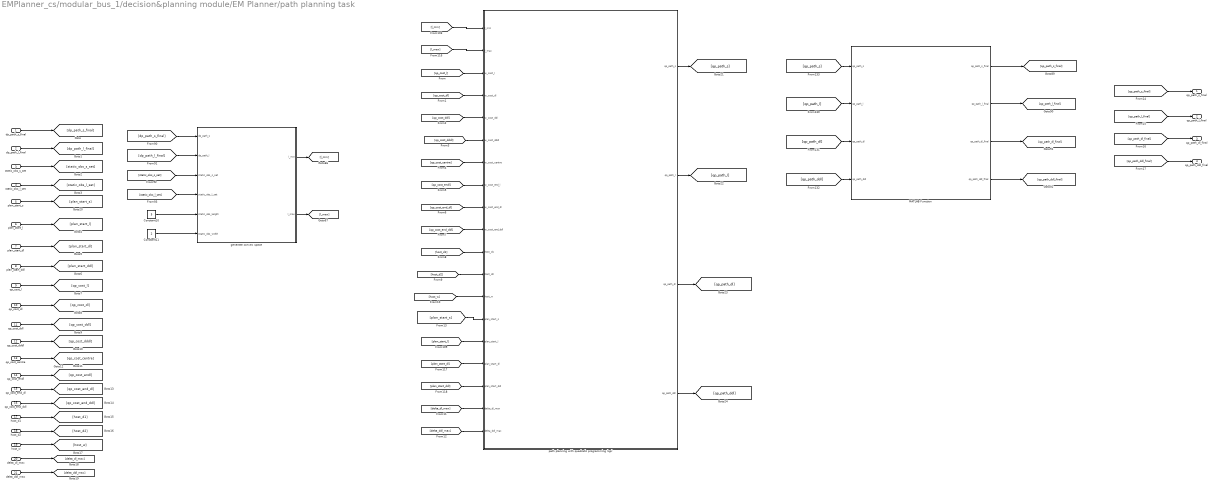
== system EMPlanner_cs/modular_bus_1/decision&planning module/EM Planner/path planning task ==
  dp_path_s_final : Inport
  dp_path_l_final : Inport  Port=2
  static_obs_s_set : Inport  Port=3
  static_obs_l_set : Inport  Port=4
  plan_start_s : Inport  Port=5
  plan_start_l : Inport  Port=6
  plan_start_dl : Inport  Port=7
  plan_start_ddl : Inport  Port=8
  qp_cost_l : Inport  Port=9
  qp_cost_dl : Inport  Port=10
  qp_cost_ddl : Inport  Port=11
  qp_cost_dddl : Inport  Port=12
  qp_cost_centre : Inport  Port=13
  qp_cost_endl : Inport  Port=14
  qp_cost_end_dl : Inport  Port=15
  qp_cost_end_ddl : Inport  Port=16
  host_d1 : Inport  Port=17
  host_d2 : Inport  Port=18
  host_w : Inport  Port=19
  delta_dl_max : Inport  Port=20
  delta_ddl_max : Inport  Port=21
  Constant10 : Constant  Value=5
  Constant11 : Constant  Value=2
  MATLAB Function : MATLAB Function  TreatAsAtomicUnit=on
  generate convex space : MATLAB Function  TreatAsAtomicUnit=on
  path planning with quadratic programming (qp) : MATLAB Function  TreatAsAtomicUnit=on
  qp_path_s_final : Outport
  qp_path_l_final : Outport  Port=2
  qp_path_dl_final : Outport  Port=3
  qp_path_ddl_final : Outport  Port=4
  wires:
  path planning with quadratic programming (qp)/4(qp_path_ddl) -> [qp_path_ddl]
  path planning with quadratic programming (qp)/3(qp_path_dl) -> [qp_path_dl]
  path planning with quadratic programming (qp)/2(qp_path_l) -> [qp_path_l]
  path planning with quadratic programming (qp)/1(qp_path_s) -> [qp_path_s]
  [qp_path_ddl_final] -> qp_path_ddl_final/1
  [qp_path_dl_final] -> qp_path_dl_final/1
  [qp_path_l_final] -> qp_path_l_final/1
  [qp_path_s_final] -> qp_path_s_final/1
  [qp_path_l] -> MATLAB Function/2(qp_path_l)
  MATLAB Function/4(qp_path_ddl_final) -> [qp_path_ddl_final]
  [qp_path_dl] -> MATLAB Function/3(qp_path_dl)
  MATLAB Function/2(qp_path_l_final) -> [qp_path_l_final]
  [qp_path_ddl] -> MATLAB Function/4(qp_path_ddl)
  [qp_path_s] -> MATLAB Function/1(qp_path_s)
  MATLAB Function/3(qp_path_dl_final) -> [qp_path_dl_final]
  MATLAB Function/1(qp_path_s_final) -> [qp_path_s_final]
  [plan_start_s] -> path planning with quadratic programming (qp)/14(plan_start_s)
  plan_start_s/1 -> [plan_start_s]
  delta_ddl_max/1 -> [delta_ddl_max]
  delta_dl_max/1 -> [delta_dl_max]
  [delta_ddl_max] -> path planning with quadratic programming (qp)/19(delta_ddl_max)
  [delta_dl_max] -> path planning with quadratic programming (qp)/18(delta_dl_max)
  host_w/1 -> [host_w]
  host_d2/1 -> [host_d2]
  host_d1/1 -> [host_d1]
  qp_cost_end_ddl/1 -> [qp_cost_end_ddl]
  qp_cost_end_dl/1 -> [qp_cost_end_dl]
  qp_cost_endl/1 -> [qp_cost_endl]
  qp_cost_centre/1 -> [qp_cost_centre]
  qp_cost_dddl/1 -> [qp_cost_dddl]
  qp_cost_ddl/1 -> [qp_cost_ddl]
  qp_cost_dl/1 -> [qp_cost_dl]
  qp_cost_l/1 -> [qp_cost_l]
  [host_w] -> path planning with quadratic programming (qp)/13(host_w)
  [host_d2] -> path planning with quadratic programming (qp)/12(host_d2)
  [host_d1] -> path planning with quadratic programming (qp)/11(host_d1)
  [qp_cost_end_ddl] -> path planning with quadratic programming (qp)/10(w_cost_end_ddl)
  [qp_cost_end_dl] -> path planning with quadratic programming (qp)/9(w_cost_end_dl)
  [qp_cost_endl] -> path planning with quadratic programming (qp)/8(w_cost_end_l)
  [qp_cost_centre] -> path planning with quadratic programming (qp)/7(w_cost_centre)
  [qp_cost_dddl] -> path planning with quadratic programming (qp)/6(w_cost_dddl)
  [qp_cost_ddl] -> path planning with quadratic programming (qp)/5(w_cost_ddl)
  [qp_cost_dl] -> path planning with quadratic programming (qp)/4(w_cost_dl)
  [qp_cost_l] -> path planning with quadratic programming (qp)/3(w_cost_l)
  plan_start_ddl/1 -> [plan_start_ddl]
  plan_start_dl/1 -> [plan_start_dl]
  plan_start_l/1 -> [plan_start_l]
  static_obs_l_set/1 -> [static_obs_l_set]
  static_obs_s_set/1 -> [static_obs_s_set]
  dp_path_l_final/1 -> [dp_path_l_final]
  dp_path_s_final/1 -> [dp_path_s_final]
  [plan_start_ddl] -> path planning with quadratic programming (qp)/17(plan_start_ddl)
  [l_min] -> path planning with quadratic programming (qp)/1(l_min)
  [l_max] -> path planning with quadratic programming (qp)/2(l_max)
  [plan_start_dl] -> path planning with quadratic programming (qp)/16(plan_start_dl)
  [dp_path_l_final] -> generate convex space/2(dp_path_l)
  [static_obs_s_set] -> generate convex space/3(static_obs_s_set)
  generate convex space/1(l_min) -> [l_min]
  [plan_start_l] -> path planning with quadratic programming (qp)/15(plan_start_l)
  [dp_path_s_final] -> generate convex space/1(dp_path_s)
  [static_obs_l_set] -> generate convex space/4(static_obs_l_set)
  Constant10/1 -> generate convex space/5(static_obs_length)
  Constant11/1 -> generate convex space/6(static_obs_width)
  generate convex space/2(l_max) -> [l_max]

== system EMPlanner_cs/modular_bus_1/control module1/control main/longitudinal control double PID/discrete pid distance ==
  err : Inport
  kp : Inport  Port=2
  ki : Inport  Port=3
  kd : Inport  Port=4
  Add2 : Sum  Inputs=+++
  Add3 : Sum
  Add4 : Sum  Inputs=+-
  Delay3 : Delay  DelayLength=1
  Delay4 : Delay  DelayLength=1
  Divide : Product  Inputs=**
  Divide1 : Product  Inputs=**
  Divide2 : Product  Inputs=**
  Gain : Gain  Gain=0.01
  pid_out : Outport
  wires:
  Gain/1 -> Delay3/1
  kd/1 -> [KD_PID_distance]
  ki/1 -> [KI_PID_distance]
  kp/1 -> [KP_PID_distance]
  Add2/1 -> pid_out/1
  Add4/1 -> Divide2/1
  [KI_PID_distance] -> Divide1/2
  Delay3/1 -> Add3/2
  Divide1/1 -> Add2/2
  [KP_PID_distance] -> Divide/1
  Delay4/1 -> Add4/2
  Add3/1 -> Divide1/1, Gain/1
  Divide2/1 -> Add2/3
  Divide/1 -> Add2/1
  err/1 -> Add4/1, Add3/1, Divide/2, Delay4/1
  [KD_PID_distance] -> Divide2/2

== system EMPlanner_cs/modular_bus_1/control module1/control main/longitudinal control double PID/discrete pid speed ==
  err : Inport
  kp : Inport  Port=2
  ki : Inport  Port=3
  kd : Inport  Port=4
  Add2 : Sum  Inputs=+++
  Add3 : Sum
  Add4 : Sum  Inputs=+-
  Delay3 : Delay  DelayLength=1
  Delay4 : Delay  DelayLength=1
  Divide : Product  Inputs=**
  Divide1 : Product  Inputs=**
  Divide2 : Product  Inputs=**
  Gain : Gain  Gain=0.01
  pid_out : Outport
  wires:
  [KD_PID_distance] -> Divide2/2
  err/1 -> Delay4/1, Divide/2, Add3/1, Add4/1
  Divide/1 -> Add2/1
  Divide2/1 -> Add2/3
  Add3/1 -> Gain/1, Divide1/1
  Delay4/1 -> Add4/2
  [KP_PID_distance] -> Divide/1
  Divide1/1 -> Add2/2
  Delay3/1 -> Add3/2
  [KI_PID_distance] -> Divide1/2
  Add4/1 -> Divide2/1
  Add2/1 -> pid_out/1
  kp/1 -> [KP_PID_distance]
  ki/1 -> [KI_PID_distance]
  kd/1 -> [KD_PID_distance]
  Gain/1 -> Delay3/1

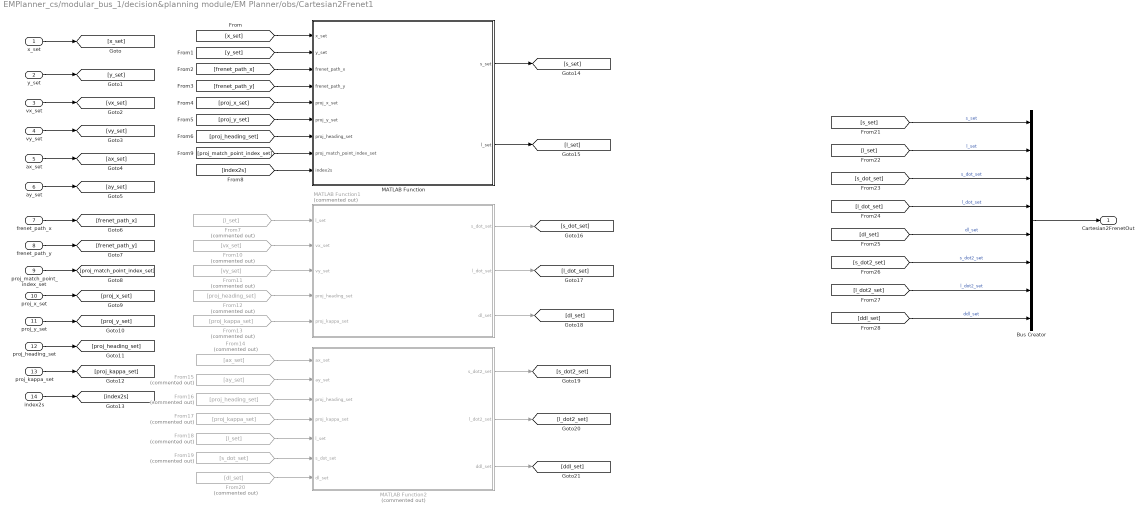
== system EMPlanner_cs/modular_bus_1/decision&planning module/EM Planner/obs/Cartesian2Frenet1 ==
  x_set : Inport
  y_set : Inport  Port=2
  vx_set : Inport  Port=3
  vy_set : Inport  Port=4
  ax_set : Inport  Port=5
  ay_set : Inport  Port=6
  frenet_path_x : Inport  Port=7
  frenet_path_y : Inport  Port=8
  proj_match_point_index_set : Inport  Port=9
  proj_x_set : Inport  Port=10
  proj_y_set : Inport  Port=11
  proj_heading_set : Inport  Port=12
  proj_kappa_set : Inport  Port=13
  index2s : Inport  Port=14
  Bus Creator : BusCreator  Inputs=8
  From10 : From  Commented=on  GotoTag=vx_set
  From11 : From  Commented=on  GotoTag=vy_set
  From12 : From  Commented=on  GotoTag=proj_heading_set
  From13 : From  Commented=on  GotoTag=proj_kappa_set
  From14 : From  Commented=on  GotoTag=ax_set
  From15 : From  Commented=on  GotoTag=ay_set
  From16 : From  Commented=on  GotoTag=proj_heading_set
  From17 : From  Commented=on  GotoTag=proj_kappa_set
  From18 : From  Commented=on  GotoTag=l_set
  From19 : From  Commented=on  GotoTag=s_dot_set
  From20 : From  Commented=on  GotoTag=dl_set
  From7 : From  Commented=on  GotoTag=l_set
  MATLAB Function : MATLAB Function  TreatAsAtomicUnit=on
  MATLAB Function1 : MATLAB Function  Commented=on  TreatAsAtomicUnit=on
  MATLAB Function2 : MATLAB Function  Commented=on  TreatAsAtomicUnit=on
  Cartesian2FrenetOut : Outport
  wires:
  x_set/1 -> [x_set]
  y_set/1 -> [y_set]
  vx_set/1 -> [vx_set]
  vy_set/1 -> [vy_set]
  ax_set/1 -> [ax_set]
  ay_set/1 -> [ay_set]
  frenet_path_x/1 -> [frenet_path_x]
  frenet_path_y/1 -> [frenet_path_y]
  proj_match_point_index_set/1 -> [proj_match_point_index_set]
  proj_x_set/1 -> [proj_x_set]
  proj_y_set/1 -> [proj_y_set]
  proj_heading_set/1 -> [proj_heading_set]
  proj_kappa_set/1 -> [proj_kappa_set]
  index2s/1 -> [index2s]
  [x_set] -> MATLAB Function/1(x_set)
  [y_set] -> MATLAB Function/2(y_set)
  [frenet_path_x] -> MATLAB Function/3(frenet_path_x)
  [frenet_path_y] -> MATLAB Function/4(frenet_path_y)
  [proj_x_set] -> MATLAB Function/5(proj_x_set)
  [proj_match_point_index_set] -> MATLAB Function/8(proj_match_point_index_set)
  [proj_y_set] -> MATLAB Function/6(proj_y_set)
  [proj_heading_set] -> MATLAB Function/7(proj_heading_set)
  [index2s] -> MATLAB Function/9(index2s)
  MATLAB Function/1(s_set) -> [s_set]
  MATLAB Function/2(l_set) -> [l_set]
  From7/1 -> MATLAB Function1/1(l_set)
  From10/1 -> MATLAB Function1/2(vx_set)
  From11/1 -> MATLAB Function1/3(vy_set)
  From12/1 -> MATLAB Function1/4(proj_heading_set)
  From13/1 -> MATLAB Function1/5(proj_kappa_set)
  From14/1 -> MATLAB Function2/1(ax_set)
  From15/1 -> MATLAB Function2/2(ay_set)
  From16/1 -> MATLAB Function2/3(proj_heading_set)
  From17/1 -> MATLAB Function2/4(proj_kappa_set)
  From18/1 -> MATLAB Function2/5(l_set)
  MATLAB Function1/1(s_dot_set) -> [s_dot_set]
  MATLAB Function1/2(l_dot_set) -> [l_dot_set]
  MATLAB Function1/3(dl_set) -> [dl_set]
  From19/1 -> MATLAB Function2/6(s_dot_set)
  From20/1 -> MATLAB Function2/7(dl_set)
  MATLAB Function2/1(s_dot2_set) -> [s_dot2_set]
  MATLAB Function2/2(l_dot2_set) -> [l_dot2_set]
  MATLAB Function2/3(ddl_set) -> [ddl_set]
  [s_set] -> Bus Creator/1  "s_set"
  [l_set] -> Bus Creator/2  "l_set"
  [s_dot_set] -> Bus Creator/3  "s_dot_set"
  [l_dot_set] -> Bus Creator/4  "l_dot_set"
  [dl_set] -> Bus Creator/5  "dl_set"
  [s_dot2_set] -> Bus Creator/6  "s_dot2_set"
  [l_dot2_set] -> Bus Creator/7  "l_dot2_set"
  [ddl_set] -> Bus Creator/8  "ddl_set"
  Bus Creator/1 -> Cartesian2FrenetOut/1

== matlab function EMPlanner_cs/modular_bus_1/control module1/control main/lateral control LQR/err_kappa_calculate_module ==
  data: x input; y input; phi input; vx input; vy input; phi_dot input; xr input; yr input; thetar input; kappar input; err output; es output; s_dot output; phi output; projection_point_thetar output
function [err,es,s_dot,phi,projection_point_thetar] = fcn(x,y,phi,vx,vy,phi_dot,xr,yr,thetar,kappar)
    
    tor=[cos(thetar);sin(thetar)];
    nor=[-sin(thetar);cos(thetar)];
    d_err=[x-xr;y-yr];
    ed=nor'*d_err;
    es=tor'*d_err;
    %projection_point_thetar=thetar(dmin);%apollo
    projection_point_thetar=thetar+kappar*es;
    ed_dot=vy*cos(phi-projection_point_thetar)+vx*sin(phi-projection_point_thetar);
    %%%%%%%%%
    ephi=sin(phi-projection_point_thetar);
    %%%%%%%%%
    ss_dot=vx*cos(phi-projection_point_thetar)-vy*sin(phi-projection_point_thetar);
    s_dot=ss_dot/(1-kappar*ed);
    ephi_dot=phi_dot-kappar*s_dot;
    err=[ed;ed_dot;ephi;ephi_dot];
    
    
    
    
    
    
    
    
    
    
    
    


end

== matlab function EMPlanner_cs/modular_bus_1/control module1/control main/lateral control LQR/feed_forword_control ==
  data: vx input; a input; forword_angle output; b input; m input; cf input; cr input; k input; kr input
function forword_angle = fcn(vx,a,b,m,cf,cr,k,kr)
    forword_angle=kr*(a+b-b*k(3)-(m*vx*vx/(a+b))*((b/cf)+(a/cr)*k(3)-(a/cr)));
end

== matlab function EMPlanner_cs/modular_bus_1/control module1/control main/lateral control LQR/feedback_control+feedforword_control ==
  data: k input; angle output; err input; forword_angle input
function angle = fcn(k,err,forword_angle)

    angle=-k*err+forword_angle;
end

== matlab function EMPlanner_cs/modular_bus_1/control module1/control main/lateral control LQR/predict_module ==
  data: x input; pred_x_ctrl output; y input; phi input; vx input; vy input; phi_dot input; ts input; pred_y_ctrl output; pred_yaw_ctrl output; pred_vx_ctrl output; pred_vy_ctrl output; pred_yaw_dot_ctrl output
function [pred_x_ctrl,pred_y_ctrl,pred_yaw_ctrl,pred_vx_ctrl,pred_vy_ctrl,pred_yaw_dot_ctrl] = fcn(x,y,phi,vx,vy,phi_dot,ts)
    pred_x_ctrl=x+vx*ts*cos(phi)-vy*ts*sin(phi);
    pred_y_ctrl=y+vy*ts*cos(phi)+vx*ts*sin(phi);
    pred_yaw_ctrl=phi;
    pred_vx_ctrl=vx;
    pred_vy_ctrl=vy;
    pred_yaw_dot_ctrl=phi_dot;
end

== matlab function EMPlanner_cs/modular_bus_1/control module1/control main/longitudinal control double PID/MATLAB Function1 ==
  data: u input; throttle output; brake output
function [throttle,brake] = fcn(u)
    if u>=0
        throttle=u;
        brake=0;
    else
        throttle=0;
        brake=-u;
    end

== matlab function EMPlanner_cs/modular_bus_1/decision&planning module/EM Planner/Cartesian2Frenet/MATLAB Function ==
  data: x_set input; s_set output; y_set input; frenet_path_x input; frenet_path_y input; proj_x_set input; proj_y_set input; proj_heading_set input; proj_match_point_index_set input; index2s input; l_set output
function [s_set,l_set] = fcn(x_set,y_set,frenet_path_x,frenet_path_y,...
    proj_x_set,proj_y_set,proj_heading_set,proj_match_point_index_set,index2s)
    %该函数将计算世界坐标系下的x_set，y_set上的点在frenet_path下的坐标s l
    %输入 x_set,y_set 待坐标转换的点
    %     frenet_path_x,frenet_path_y   frenet坐标轴
    %     proj_x,y,heading,kappa,proj_match_point_index 待坐标转换的点的投影点的信息
    %     index2s   frenet_path的index与s的转换表

    % 由于不知道有多少个点需要做坐标转换，所以需要做缓冲
    n = 128;%最多处理128个点
    %输出初始化
    s_set = ones(n,1)*nan;
    l_set = ones(n,1)*nan;
    for i = 1:length(x_set)
        if isnan(x_set(i))
            break;
        end
        %计算s，写个子函数
        s_set(i) = CalcSFromIndex2S(index2s,frenet_path_x,frenet_path_y,proj_x_set(i),proj_y_set(i),...
            proj_match_point_index_set(i));
        n_r = [-sin(proj_heading_set(i));cos(proj_heading_set(i))];
        r_h = [x_set(i);y_set(i)];
        r_r = [proj_x_set(i);proj_y_set(i)];
        l_set(i) = (r_h - r_r)'*n_r;
    end
end

function s = CalcSFromIndex2S(index2s,path_x,path_y,proj_x,proj_y,proj_match_point_index)
  %该函数将计算当指定index2s的映射关系后，计算点proj_x,proj_y的弧长
  vector_1 = [proj_x;proj_y] - [path_x(proj_match_point_index);path_y(proj_match_point_index)];
  %这里要考虑的更全面一些，因为要考虑到proj_match_point_index有可能在path的起点或终点
  if (proj_match_point_index < length(path_x))
      vector_2 = [path_x(proj_match_point_index + 1);path_y(proj_match_point_index + 1)] - ...
          [path_x(proj_match_point_index);path_y(proj_match_point_index)];
  else
      vector_2 = [path_x(proj_match_point_index);path_y(proj_match_point_index)] - ...
          [path_x(proj_match_point_index - 1);path_y(proj_match_point_index - 1)];
  end
  
  if vector_1'*vector_2 > 0
      s = index2s(proj_match_point_index) + sqrt(vector_1'*vector_1);
  else
      s = index2s(proj_match_point_index) - sqrt(vector_1'*vector_1);
  end
  
  
end

== matlab function EMPlanner_cs/modular_bus_1/decision&planning module/EM Planner/Cartesian2Frenet/MATLAB Function1 ==
  data: l_set input; s_dot_set output; vx_set input; vy_set input; proj_heading_set input; proj_kappa_set input; l_dot_set output; dl_set output
function [s_dot_set,l_dot_set,dl_set] = fcn(l_set,vx_set,vy_set,proj_heading_set,proj_kappa_set)
%该函数将计算frenet坐标系下的s_dot, l_dot, dl/ds
n = 128;
% 输出初始化
s_dot_set = ones(n,1)*nan;
l_dot_set = ones(n,1)*nan;
dl_set = ones(n,1)*nan;

for i = 1 : length(l_set)
    if isnan(l_set(i))
        break;
    end
    v_h = [vx_set(i);vy_set(i)];
    n_r = [-sin(proj_heading_set(i));cos(proj_heading_set(i))];
    t_r = [cos(proj_heading_set(i));sin(proj_heading_set(i))];
    l_dot_set(i) = v_h'*n_r;
    s_dot_set(i) = v_h'*t_r/(1 - proj_kappa_set(i)*l_set(i));
    %%%向量法做cartesian与frenet的转换要更简单，但是也有缺点，向量法必须依赖速度加速度
    %l' = l_dot/s_dot 但是如果s_dot = 0 此方法就失效了
    if abs(s_dot_set(i)) < 1e-6
        dl_set(i) = 0;
    else
        dl_set(i) = l_dot_set(i)/s_dot_set(i);
    end
end

== matlab function EMPlanner_cs/modular_bus_1/decision&planning module/EM Planner/Cartesian2Frenet/MATLAB Function2 ==
  data: ax_set input; s_dot2_set output; ay_set input; proj_heading_set input; proj_kappa_set input; l_set input; s_dot_set input; dl_set input; l_dot2_set output; ddl_set output
function [s_dot2_set,l_dot2_set,ddl_set] = fcn(ax_set,ay_set,proj_heading_set,proj_kappa_set,l_set,s_dot_set,dl_set)
%由于不知道有多少个点需要做坐标转换，设一个最大值做缓冲
n = 128;
% 输出初始化
s_dot2_set = ones(n,1)*nan;
l_dot2_set = ones(n,1)*nan;
ddl_set = ones(n,1)*nan;

for i = 1:length(l_set)
    if isnan(l_set(i))
       break;
    end
    a_h = [ax_set(i);ay_set(i)];
    n_r = [-sin(proj_heading_set(i));cos(proj_heading_set(i))];
    t_r = [cos(proj_heading_set(i));sin(proj_heading_set(i))];
    %近似认为dkr/ds 为0 简化计算
    l_dot2_set(i) = a_h'*n_r - proj_kappa_set(i) * (1 - proj_kappa_set(i) * l_set(i)) * s_dot_set(i)^2;
    s_dot2_set(i) = (1/(1 - proj_kappa_set(i) * l_set(i)))* (a_h' * t_r + 2 * proj_kappa_set(i) * dl_set(i) * s_dot_set(i)^2);
    % 要考虑加速度为0的情况
    if (s_dot2_set(i) < 1e-6)
        ddl_set(i) = 0;
    else
        ddl_set(i) = (l_dot2_set(i) - dl_set(i)*s_dot2_set(i))/(s_dot_set(i)^2);
    end
end

== matlab function EMPlanner_cs/modular_bus_1/decision&planning module/EM Planner/Cartesian2Frenet1/MATLAB Function ==
  data: x_set input; s_set output; y_set input; frenet_path_x input; frenet_path_y input; proj_x_set input; proj_y_set input; proj_heading_set input; proj_match_point_index_set input; index2s input; l_set output
function [s_set,l_set] = fcn(x_set,y_set,frenet_path_x,frenet_path_y,...
    proj_x_set,proj_y_set,proj_heading_set,proj_match_point_index_set,index2s)
    %该函数将计算世界坐标系下的x_set，y_set上的点在frenet_path下的坐标s l
    %输入 x_set,y_set 待坐标转换的点
    %     frenet_path_x,frenet_path_y   frenet坐标轴
    %     proj_x,y,heading,kappa,proj_match_point_index 待坐标转换的点的投影点的信息
    %     index2s   frenet_path的index与s的转换表

    % 由于不知道有多少个点需要做坐标转换，所以需要做缓冲
    n = 128;%最多处理128个点
    %输出初始化
    s_set = ones(n,1)*nan;
    l_set = ones(n,1)*nan;
    for i = 1:length(x_set)
        if isnan(x_set(i))
            break;
        end
        %计算s，写个子函数
        s_set(i) = CalcSFromIndex2S(index2s,frenet_path_x,frenet_path_y,proj_x_set(i),proj_y_set(i),...
            proj_match_point_index_set(i));
        n_r = [-sin(proj_heading_set(i));cos(proj_heading_set(i))];
        r_h = [x_set(i);y_set(i)];
        r_r = [proj_x_set(i);proj_y_set(i)];
        l_set(i) = (r_h - r_r)'*n_r;
    end
end

function s = CalcSFromIndex2S(index2s,path_x,path_y,proj_x,proj_y,proj_match_point_index)
  %该函数将计算当指定index2s的映射关系后，计算点proj_x,proj_y的弧长
  vector_1 = [proj_x;proj_y] - [path_x(proj_match_point_index);path_y(proj_match_point_index)];
  %这里要考虑的更全面一些，因为要考虑到proj_match_point_index有可能在path的起点或终点
  if (proj_match_point_index < length(path_x))
      vector_2 = [path_x(proj_match_point_index + 1);path_y(proj_match_point_index + 1)] - ...
          [path_x(proj_match_point_index);path_y(proj_match_point_index)];
  else
      vector_2 = [path_x(proj_match_point_index);path_y(proj_match_point_index)] - ...
          [path_x(proj_match_point_index - 1);path_y(proj_match_point_index - 1)];
  end
  
  if vector_1'*vector_2 > 0
      s = index2s(proj_match_point_index) + sqrt(vector_1'*vector_1);
  else
      s = index2s(proj_match_point_index) - sqrt(vector_1'*vector_1);
  end
  
  
end

== matlab function EMPlanner_cs/modular_bus_1/decision&planning module/EM Planner/Cartesian2Frenet1/MATLAB Function1 ==
  data: l_set input; s_dot_set output; vx_set input; vy_set input; proj_heading_set input; proj_kappa_set input; l_dot_set output; dl_set output
function [s_dot_set,l_dot_set,dl_set] = fcn(l_set,vx_set,vy_set,proj_heading_set,proj_kappa_set)
%该函数将计算frenet坐标系下的s_dot, l_dot, dl/ds
n = 128;
% 输出初始化
s_dot_set = ones(n,1)*nan;
l_dot_set = ones(n,1)*nan;
dl_set = ones(n,1)*nan;

for i = 1 : length(l_set)
    if isnan(l_set(i))
        break;
    end
    v_h = [vx_set(i);vy_set(i)];
    n_r = [-sin(proj_heading_set(i));cos(proj_heading_set(i))];
    t_r = [cos(proj_heading_set(i));sin(proj_heading_set(i))];
    l_dot_set(i) = v_h'*n_r;
    s_dot_set(i) = v_h'*t_r/(1 - proj_kappa_set(i)*l_set(i));
    %%%向量法做cartesian与frenet的转换要更简单，但是也有缺点，向量法必须依赖速度加速度
    %l' = l_dot/s_dot 但是如果s_dot = 0 此方法就失效了
    if abs(s_dot_set(i)) < 1e-6
        dl_set(i) = 0;
    else
        dl_set(i) = l_dot_set(i)/s_dot_set(i);
    end
end

== matlab function EMPlanner_cs/modular_bus_1/decision&planning module/EM Planner/Cartesian2Frenet1/MATLAB Function2 ==
  data: ax_set input; s_dot2_set output; ay_set input; proj_heading_set input; proj_kappa_set input; l_set input; s_dot_set input; dl_set input; l_dot2_set output; ddl_set output
function [s_dot2_set,l_dot2_set,ddl_set] = fcn(ax_set,ay_set,proj_heading_set,proj_kappa_set,l_set,s_dot_set,dl_set)
%由于不知道有多少个点需要做坐标转换，设一个最大值做缓冲
n = 128;
% 输出初始化
s_dot2_set = ones(n,1)*nan;
l_dot2_set = ones(n,1)*nan;
ddl_set = ones(n,1)*nan;

for i = 1:length(l_set)
    if isnan(l_set(i))
       break;
    end
    a_h = [ax_set(i);ay_set(i)];
    n_r = [-sin(proj_heading_set(i));cos(proj_heading_set(i))];
    t_r = [cos(proj_heading_set(i));sin(proj_heading_set(i))];
    %近似认为dkr/ds 为0 简化计算
    l_dot2_set(i) = a_h'*n_r - proj_kappa_set(i) * (1 - proj_kappa_set(i) * l_set(i)) * s_dot_set(i)^2;
    s_dot2_set(i) = (1/(1 - proj_kappa_set(i) * l_set(i)))* (a_h' * t_r + 2 * proj_kappa_set(i) * dl_set(i) * s_dot_set(i)^2);
    % 要考虑加速度为0的情况
    if (s_dot2_set(i) < 1e-6)
        ddl_set(i) = 0;
    else
        ddl_set(i) = (l_dot2_set(i) - dl_set(i)*s_dot2_set(i))/(s_dot_set(i)^2);
    end
end
